simulink model "GFMGSP"  (R2022a)
settings: Solver=FixedStepAuto  StartTime=0.0  StopTime=3  FixedStep=Ts  RelTol=1e-3
values from neighbouring files (symbols this model uses):
  Cf1 = 0.002    [GFMGSP_Para.m]
  Cf2 = 0.2    [GFMGSP_Para.m]
  dt_jump = 2    [GFMGSP_Para.m]
  dt_sag = 0.01    [GFMGSP_Para.m]
  ki_pll1 = 0    [GFMGSP_Para.m]
  kp_pll1 = w_pll1    [GFMGSP_Para.m]
  Kq = Kq    [GFMGSP_Para.m]
  L1 = X1    [GFMGSP_Para.m]
  L2 = X2    [GFMGSP_Para.m]
  Lc1 = 1e-9    (= 1e-09)    [GFMGSP_Para.m]
  Lc2 = 1e-9    (= 1e-09)    [GFMGSP_Para.m]
  Lf1 = 0.1    [GFMGSP_Para.m]
  Lf2 = 0.1    [GFMGSP_Para.m]
  Lg = Xg    [GFMGSP_Para.m]
  M = Kgfm/Wbase    [GFMGSP_Para.m]
  phase_jump = -1.2    [GFMGSP_Para.m]
  Pm = Pref    [GFMGSP_Para.m]
  position = position    [GFMGSP_Para.m]
  R1 = R1    [GFMGSP_Para.m]
  R2 = R2    [GFMGSP_Para.m]
  Rg = Rg    [GFMGSP_Para.m]
  Sbase = 1    [GFMGSP_Para.m]
  Scale_ki_v = 60    [GFMGSP_Para.m]
  t0 = 2    [GFMGSP_Para.m]
  t0_jump = 10    [GFMGSP_Para.m]
  t0_sag = 10    [GFMGSP_Para.m]
  tc1 = t_c-0.002    [GFMGSP_Para.m]
  tc2 = t_c2    [GFMGSP_Para.m]
  tc3 = t_c3    [GFMGSP_Para.m]
  Ts = 1/Fs    (= 1e-05)    [GFMGSP_Para.m]
  v_sag = 0.1    [GFMGSP_Para.m]
  Vbase = 1    [GFMGSP_Para.m]
  w_droop = 15*2*pi    (= 94.2477796077)    [GFMGSP_Para.m]
  w_i_GFL1 = 1000 *2*pi    (= 6283.18530718)    [GFMGSP_Para.m]
  w_i_GFM = 2500*2*pi    (= 15707.9632679)    [GFMGSP_Para.m]
  w_pll1 = k1p    [GFMGSP_Para.m]
  w_tau1 = 1e3 *2*pi    (= 6283.18530718)    [GFMGSP_Para.m]
  w_tvc = 25*2*pi    (= 157.079632679)    [GFMGSP_Para.m]
  w_v_GFM = 200 *2*pi    (= 1256.63706144)    [GFMGSP_Para.m]
  Wbase = 2*pi*50    (= 314.159265359)    [GFMGSP_Para.m]
  Zbase = Vbase/Ibase    (= 1)    [GFMGSP_Para.m]
undefined symbols (not defined in the file or in its folder): DiscIntNeverNeededParam, I1d, I1q, initial, V1ref
libraries: spsVoltageMeasurementLib x114, spsCurrentMeasurementLib x93, spsThreePhaseSeriesRLCBranchLib x45, SimplexPS x42, spsControlledVoltageSourceLib x39, SimplexPS_2015a x14, spsGroundLib x10, spsSeriesRLCBranchLib x9, spsThreePhaseBreakerLib x6, spsMultimeterLib x3, spsThreePhaseFaultLib x3, spspowerguiLib x1
(part 3 of 7)

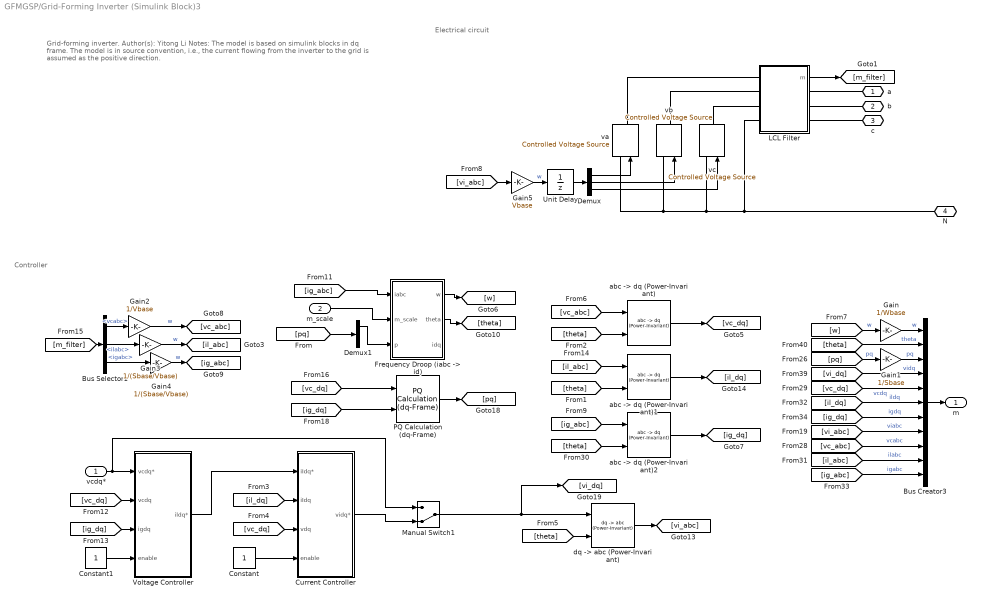
== system GFMGSP/Grid-Forming Inverter (Simulink Block)3 ==
  note: Grid-forming inverter.
      |
      | Author(s): Yitong Li
      |
      | Notes:
      |
      | The model is based on simulink blocks in dq frame.
      |
      | The model is in source convention, i.e., the current flowing from the inverter to the grid is assumed as the positive direction.
  note: Electrical circuit
  note: Controller
  vcdq* : Inport
  m_scale : Inport  Port=2
  Bus Creator3 : BusCreator  Inputs=11
  Bus Selector1 : BusSelector  OutputSignals=vcabc,ilabc,igabc
  Constant : Constant
  Constant1 : Constant
  Current Controller : Subsystem  mask{Ts=Ts, Wbase=Wbase, Lf=Lf/Wbase, Kg=0, Kp=w_i*Lf/Wbase, Ki=w_i*w_i/4*Lf/Wbase, xdmax=inf, xqmax=inf, Kcd=0}
      mask prompts: Ts "Sampling Time (s)"; Wbase "Base Angular Frequency (rad/s)"; Lf "Inductance"; Kg "Estimator Gain"; Kp "Proportional Gain"; Ki "Integral Gain"; xdmax "Voltage D Limit"; xqmax "Voltage Q Limit"; Kcd "Cross Decoupling Gain"
  Demux : Demux  Outputs=3
  Demux1 : Demux  Outputs=2
  "Frequency Droop (iabc -> id)" : Subsystem  AncestorBlock=|  mask{Ts=Ts, Sbase=Sbase, Vbase=Vbase, Wbase=Wbase, m=m, w_tau=w_droop, theta0=0, i0=Pm, w0=1}
      | SimplexPS/Frequency Droop
      | (iabc -> id)
      mask prompts: Ts "Ts (s), samping period"; Sbase "Sbase (VA), base power"; Vbase "Vbase (V), base voltage"; Wbase "Wbase (rad/s), base angular frequency"; m "m (pu), droop gain"; w_tau "w_tau (rad/s), low-pass filter bandwidth"; theta0 "theta0 (rad), initial angle"; i0 "i0 (pu), current setting point"; w0 "w0 (pu), frequency setting point"
  Gain : Gain  Gain=1/Wbase
  Gain1 : Gain  Gain=1/Sbase
  Gain2 : Gain  Gain=1/Vbase
  Gain3 : Gain  Gain=1/(Sbase/Vbase)
  Gain4 : Gain  Gain=1/(Sbase/Vbase)
  Gain5 : Gain  Gain=Vbase
  LCL Filter : Subsystem  AncestorBlock=SimplexPS/LCL Filter  mask{Lf=Lf*(Vbase^2/Sbase)/Wbase, Rf=1e-2*(Vbase^2/Sbase), Lc=Lc*(Vbase^2/Sbase)/Wbase, Rc=1e-9*(Vbase^2/Sbase), Cf=Cf*(Sbase/Vbase^2)/Wbase, Rd=1e-3*(Vbase^2/Sbase)}
      mask prompts: Lf "Lf (H)"; Rf "Rf (Ohm)"; Lc "Lc (H)"; Rc "Rc (Ohm)"; Cf "Cf (F)"; Rd "Rd (Ohm)"
  Manual Switch1 : ManualSwitch  CurrentSetting=0
  PQ Calculation (dq-Frame) : SimplexPS/PQ Calculation (dq-Frame)  SystemSampleTime=-1  VariantActivationTime=update diagram  Latency=0  AutoFrameSizeCalculation=off
      settings: SourceProductName=Simplex Power Systems
  Unit Delay : UnitDelay  SampleTime=-1  HasFrameUpgradeWarning=on
  Voltage Controller : Subsystem  mask{Ts=Ts, Wbase=Wbase, Cf=Cf/Wbase, Kg=0, Kp=w_v*Cf/Wbase, Ki=w_v*w_v/4*Cf/Wbase*Scale_ki_v, xdmax=inf, xqmax=inf, Kcd=0}
      mask prompts: Ts "Sampling Time (s)"; Wbase "Base Angular Frequency (rad/s)"; Cf "Capacitance"; Kg "Estimator Gain"; Kp "Proportional Gain"; Ki "Integral Gain"; xdmax "Current D Limit"; xqmax "Current Q Limit"; Kcd "Cross Decoupling Gain"
  "abc -> dq (Power-Invariant)" : SimplexPS/abc -> dq (Power-Invariant)  SystemSampleTime=-1  VariantActivationTime=update diagram  Latency=0  AutoFrameSizeCalculation=off
      settings: SourceProductName=Simplex Power Systems
  "abc -> dq (Power-Invariant)1" : SimplexPS/abc -> dq (Power-Invariant)  SystemSampleTime=-1  VariantActivationTime=update diagram  Latency=0  AutoFrameSizeCalculation=off
      settings: SourceProductName=Simplex Power Systems
  "abc -> dq (Power-Invariant)2" : SimplexPS/abc -> dq (Power-Invariant)  SystemSampleTime=-1  VariantActivationTime=update diagram  Latency=0  AutoFrameSizeCalculation=off
      settings: SourceProductName=Simplex Power Systems
  "dq -> abc (Power-Invariant)" : SimplexPS/dq -> abc (Power-Invariant)  SystemSampleTime=-1  VariantActivationTime=update diagram  Latency=0  AutoFrameSizeCalculation=off
      settings: SourceProductName=Simplex Power Systems
  va : spsControlledVoltageSourceLib/Controlled Voltage Source  Initialize=on  Source_Type=AC  Amplitude=0  Phase=0  Frequency=0  Measurements=None
  vb : spsControlledVoltageSourceLib/Controlled Voltage Source  Initialize=on  Source_Type=AC  Amplitude=0  Phase=0  Frequency=0  Measurements=None
  vc : spsControlledVoltageSourceLib/Controlled Voltage Source  Initialize=on  Source_Type=AC  Amplitude=0  Phase=0  Frequency=0  Measurements=None
  a : PMIOPort  Side=Right
  b : PMIOPort  Port=2  Side=Right
  c : PMIOPort  Port=3  Side=Right
  N : PMIOPort  Port=4  Side=Right
  m : Outport
  wires:
  [ig_dq] -> Voltage Controller/3(igdq)
  [vc_dq] -> Voltage Controller/2(vcdq)
  Constant1/1 -> Voltage Controller/4(enable)
  Voltage Controller/1(ildq*) -> Current Controller/1(iIdq*)
  vcdq*/1 -> Manual Switch1/1, Voltage Controller/1(vcdq*)
  [ig_abc] -> Bus Creator3/11  "igabc"
  [il_abc] -> Bus Creator3/10  "ilabc"
  [vc_abc] -> Bus Creator3/9  "vcabc"
  [vi_abc] -> Bus Creator3/8  "viabc"
  [ig_dq] -> Bus Creator3/7  "igdq"
  [il_dq] -> Bus Creator3/6  "ildq"
  [vc_dq] -> Bus Creator3/5  "vcdq"
  [vi_dq] -> Bus Creator3/4  "vidq"
  Gain1/1 -> Bus Creator3/3  "pq"
  [theta] -> Bus Creator3/2  "theta"
  Gain/1 -> Bus Creator3/1  "w"
  [pq] -> Gain1/1  "pq"
  [w] -> Gain/1  "w"
  "abc -> dq (Power-Invariant)1"/1 -> [il_dq]
  "abc -> dq (Power-Invariant)2"/1 -> [ig_dq]
  "abc -> dq (Power-Invariant)"/1 -> [vc_dq]
  [ig_abc] -> "Frequency Droop (iabc -> id)"/1(iabc)
  [il_dq] -> Current Controller/2(iIdq)
  [ig_dq] -> PQ Calculation (dq-Frame)/2
  PQ Calculation (dq-Frame)/1 -> [pq]
  [vc_dq] -> PQ Calculation (dq-Frame)/1
  [theta] -> "dq -> abc (Power-Invariant)"/2
  [vc_dq] -> Current Controller/3(vdq)
  Constant/1 -> Current Controller/4(enable)
  "Frequency Droop (iabc -> id)"/1(w) -> [w]
  "Frequency Droop (iabc -> id)"/2(theta) -> [theta]
  [theta] -> "abc -> dq (Power-Invariant)2"/2
  [ig_abc] -> "abc -> dq (Power-Invariant)2"/1
  [il_abc] -> "abc -> dq (Power-Invariant)1"/1
  [vc_abc] -> "abc -> dq (Power-Invariant)"/1
  [theta] -> "abc -> dq (Power-Invariant)1"/2
  [theta] -> "abc -> dq (Power-Invariant)"/2
  Demux/3 -> vc/1
  Demux/2 -> vb/1
  Demux/1 -> va/1
  LCL Filter/1(m) -> [m_filter]
  Bus Creator3/1 -> m/1
  "dq -> abc (Power-Invariant)"/1 -> [vi_abc]
  m_scale/1 -> "Frequency Droop (iabc -> id)"/2(m_scale)
  [vi_abc] -> Gain5/1
  Unit Delay/1 -> Demux/1
  Demux1/1 -> "Frequency Droop (iabc -> id)"/3(p)
  [pq] -> Demux1/1
  Bus Selector1/3 -> Gain4/1  "<igabc>"
  Bus Selector1/2 -> Gain3/1  "<ilabc>"
  Bus Selector1/1 -> Gain2/1  "<vcabc>"
  Gain4/1 -> [ig_abc]  "w"
  [m_filter] -> Bus Selector1/1
  Gain2/1 -> [vc_abc]  "w"
  Gain3/1 -> [il_abc]  "w"
  Gain5/1 -> Unit Delay/1  "w"
  Manual Switch1/1 -> [vi_dq], "dq -> abc (Power-Invariant)"/1
  Current Controller/1(vidq*) -> Manual Switch1/2
  connections:
  LCL Filter/LConn3 -- vc/RConn1
  va/LConn1 -- vb/LConn1 -- vc/LConn1 -- LCL Filter/LConn4 -- N/RConn1
  LCL Filter/RConn3 -- c/RConn1
  LCL Filter/RConn2 -- b/RConn1
  LCL Filter/RConn1 -- a/RConn1
  LCL Filter/LConn1 -- va/RConn1
  LCL Filter/LConn2 -- vb/RConn1

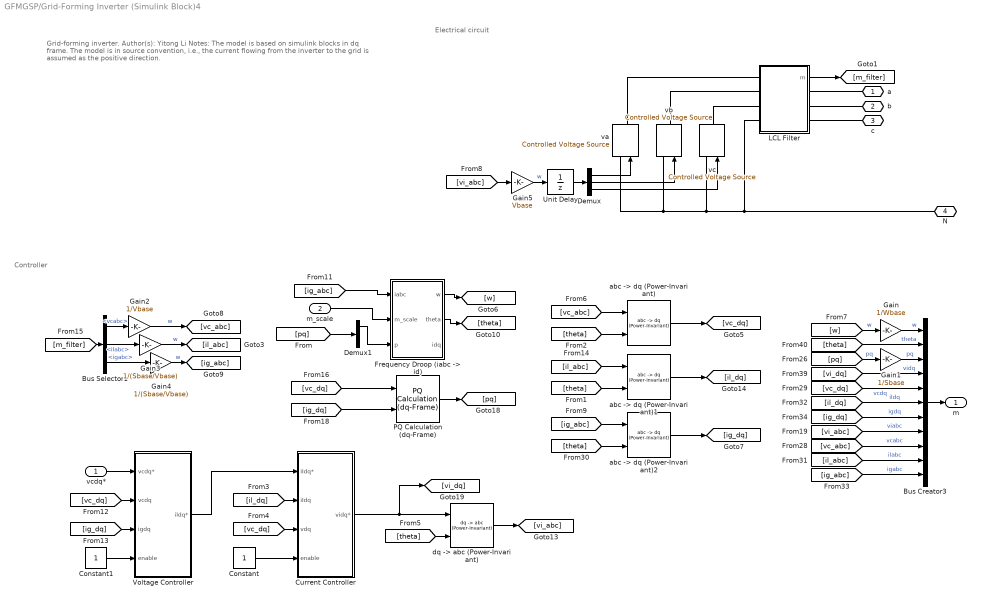
== system GFMGSP/Grid-Forming Inverter (Simulink Block)4 ==
  note: Grid-forming inverter.
      |
      | Author(s): Yitong Li
      |
      | Notes:
      |
      | The model is based on simulink blocks in dq frame.
      |
      | The model is in source convention, i.e., the current flowing from the inverter to the grid is assumed as the positive direction.
  note: Electrical circuit
  note: Controller
  vcdq* : Inport
  m_scale : Inport  Port=2
  Bus Creator3 : BusCreator  Inputs=11
  Bus Selector1 : BusSelector  OutputSignals=vcabc,ilabc,igabc
  Constant : Constant
  Constant1 : Constant
  Current Controller : Subsystem  mask{Ts=Ts, Wbase=Wbase, Lf=Lf/Wbase, Kg=0, Kp=w_i*Lf/Wbase, Ki=w_i*w_i/4*Lf/Wbase, xdmax=inf, xqmax=inf, Kcd=0}
      mask prompts: Ts "Sampling Time (s)"; Wbase "Base Angular Frequency (rad/s)"; Lf "Inductance"; Kg "Estimator Gain"; Kp "Proportional Gain"; Ki "Integral Gain"; xdmax "Voltage D Limit"; xqmax "Voltage Q Limit"; Kcd "Cross Decoupling Gain"
  Demux : Demux  Outputs=3
  Demux1 : Demux  Outputs=2
  "Frequency Droop (iabc -> id)" : Subsystem  AncestorBlock=|  mask{Ts=Ts, Sbase=Sbase, Vbase=Vbase, Wbase=Wbase, m=m, w_tau=w_droop, theta0=0, i0=Pm, w0=1}
      | SimplexPS/Frequency Droop
      | (iabc -> id)
      mask prompts: Ts "Ts (s), samping period"; Sbase "Sbase (VA), base power"; Vbase "Vbase (V), base voltage"; Wbase "Wbase (rad/s), base angular frequency"; m "m (pu), droop gain"; w_tau "w_tau (rad/s), low-pass filter bandwidth"; theta0 "theta0 (rad), initial angle"; i0 "i0 (pu), current setting point"; w0 "w0 (pu), frequency setting point"
  Gain : Gain  Gain=1/Wbase
  Gain1 : Gain  Gain=1/Sbase
  Gain2 : Gain  Gain=1/Vbase
  Gain3 : Gain  Gain=1/(Sbase/Vbase)
  Gain4 : Gain  Gain=1/(Sbase/Vbase)
  Gain5 : Gain  Gain=Vbase
  LCL Filter : Subsystem  AncestorBlock=SimplexPS/LCL Filter  mask{Lf=Lf*(Vbase^2/Sbase)/Wbase, Rf=1e-9*(Vbase^2/Sbase), Lc=Lc*(Vbase^2/Sbase)/Wbase, Rc=1e-9*(Vbase^2/Sbase), Cf=Cf*(Sbase/Vbase^2)/Wbase, Rd=1e-9*(Vbase^2/Sbase)}
      mask prompts: Lf "Lf (H)"; Rf "Rf (Ohm)"; Lc "Lc (H)"; Rc "Rc (Ohm)"; Cf "Cf (F)"; Rd "Rd (Ohm)"
  PQ Calculation (dq-Frame) : SimplexPS/PQ Calculation (dq-Frame)  SystemSampleTime=-1  VariantActivationTime=update diagram  Latency=0  AutoFrameSizeCalculation=off
      settings: SourceProductName=Simplex Power Systems
  Unit Delay : UnitDelay  SampleTime=-1  HasFrameUpgradeWarning=on
  Voltage Controller : Subsystem  mask{Ts=Ts, Wbase=Wbase, Cf=Cf/Wbase, Kg=0, Kp=w_v*Cf/Wbase, Ki=w_v*w_v/4*Cf/Wbase*Scale_ki_v, xdmax=inf, xqmax=inf, Kcd=0}
      mask prompts: Ts "Sampling Time (s)"; Wbase "Base Angular Frequency (rad/s)"; Cf "Capacitance"; Kg "Estimator Gain"; Kp "Proportional Gain"; Ki "Integral Gain"; xdmax "Current D Limit"; xqmax "Current Q Limit"; Kcd "Cross Decoupling Gain"
  "abc -> dq (Power-Invariant)" : SimplexPS/abc -> dq (Power-Invariant)  SystemSampleTime=-1  VariantActivationTime=update diagram  Latency=0  AutoFrameSizeCalculation=off
      settings: SourceProductName=Simplex Power Systems
  "abc -> dq (Power-Invariant)1" : SimplexPS/abc -> dq (Power-Invariant)  SystemSampleTime=-1  VariantActivationTime=update diagram  Latency=0  AutoFrameSizeCalculation=off
      settings: SourceProductName=Simplex Power Systems
  "abc -> dq (Power-Invariant)2" : SimplexPS/abc -> dq (Power-Invariant)  SystemSampleTime=-1  VariantActivationTime=update diagram  Latency=0  AutoFrameSizeCalculation=off
      settings: SourceProductName=Simplex Power Systems
  "dq -> abc (Power-Invariant)" : SimplexPS/dq -> abc (Power-Invariant)  SystemSampleTime=-1  VariantActivationTime=update diagram  Latency=0  AutoFrameSizeCalculation=off
      settings: SourceProductName=Simplex Power Systems
  va : spsControlledVoltageSourceLib/Controlled Voltage Source  Initialize=on  Source_Type=AC  Amplitude=0  Phase=0  Frequency=0  Measurements=None
  vb : spsControlledVoltageSourceLib/Controlled Voltage Source  Initialize=on  Source_Type=AC  Amplitude=0  Phase=0  Frequency=0  Measurements=None
  vc : spsControlledVoltageSourceLib/Controlled Voltage Source  Initialize=on  Source_Type=AC  Amplitude=0  Phase=0  Frequency=0  Measurements=None
  a : PMIOPort  Side=Right
  b : PMIOPort  Port=2  Side=Right
  c : PMIOPort  Port=3  Side=Right
  N : PMIOPort  Port=4  Side=Right
  m : Outport
  wires:
  [ig_dq] -> Voltage Controller/3(igdq)
  [vc_dq] -> Voltage Controller/2(vcdq)
  Constant1/1 -> Voltage Controller/4(enable)
  Voltage Controller/1(ildq*) -> Current Controller/1(iIdq*)
  vcdq*/1 -> Voltage Controller/1(vcdq*)
  [ig_abc] -> Bus Creator3/11  "igabc"
  [il_abc] -> Bus Creator3/10  "ilabc"
  [vc_abc] -> Bus Creator3/9  "vcabc"
  [vi_abc] -> Bus Creator3/8  "viabc"
  [ig_dq] -> Bus Creator3/7  "igdq"
  [il_dq] -> Bus Creator3/6  "ildq"
  [vc_dq] -> Bus Creator3/5  "vcdq"
  [vi_dq] -> Bus Creator3/4  "vidq"
  Gain1/1 -> Bus Creator3/3  "pq"
  [theta] -> Bus Creator3/2  "theta"
  Gain/1 -> Bus Creator3/1  "w"
  [pq] -> Gain1/1  "pq"
  [w] -> Gain/1  "w"
  "abc -> dq (Power-Invariant)1"/1 -> [il_dq]
  "abc -> dq (Power-Invariant)2"/1 -> [ig_dq]
  "abc -> dq (Power-Invariant)"/1 -> [vc_dq]
  [ig_abc] -> "Frequency Droop (iabc -> id)"/1(iabc)
  [il_dq] -> Current Controller/2(iIdq)
  [ig_dq] -> PQ Calculation (dq-Frame)/2
  PQ Calculation (dq-Frame)/1 -> [pq]
  [vc_dq] -> PQ Calculation (dq-Frame)/1
  [theta] -> "dq -> abc (Power-Invariant)"/2
  Current Controller/1(vidq*) -> "dq -> abc (Power-Invariant)"/1, [vi_dq]
  [vc_dq] -> Current Controller/3(vdq)
  Constant/1 -> Current Controller/4(enable)
  "Frequency Droop (iabc -> id)"/1(w) -> [w]
  "Frequency Droop (iabc -> id)"/2(theta) -> [theta]
  [theta] -> "abc -> dq (Power-Invariant)2"/2
  [ig_abc] -> "abc -> dq (Power-Invariant)2"/1
  [il_abc] -> "abc -> dq (Power-Invariant)1"/1
  [vc_abc] -> "abc -> dq (Power-Invariant)"/1
  [theta] -> "abc -> dq (Power-Invariant)1"/2
  [theta] -> "abc -> dq (Power-Invariant)"/2
  Demux/3 -> vc/1
  Demux/2 -> vb/1
  Demux/1 -> va/1
  LCL Filter/1(m) -> [m_filter]
  Bus Creator3/1 -> m/1
  "dq -> abc (Power-Invariant)"/1 -> [vi_abc]
  m_scale/1 -> "Frequency Droop (iabc -> id)"/2(m_scale)
  [vi_abc] -> Gain5/1
  Unit Delay/1 -> Demux/1
  Demux1/1 -> "Frequency Droop (iabc -> id)"/3(p)
  [pq] -> Demux1/1
  Bus Selector1/3 -> Gain4/1  "<igabc>"
  Bus Selector1/2 -> Gain3/1  "<ilabc>"
  Bus Selector1/1 -> Gain2/1  "<vcabc>"
  Gain4/1 -> [ig_abc]  "w"
  [m_filter] -> Bus Selector1/1
  Gain2/1 -> [vc_abc]  "w"
  Gain3/1 -> [il_abc]  "w"
  Gain5/1 -> Unit Delay/1  "w"
  connections:
  LCL Filter/LConn3 -- vc/RConn1
  va/LConn1 -- vb/LConn1 -- vc/LConn1 -- LCL Filter/LConn4 -- N/RConn1
  LCL Filter/RConn3 -- c/RConn1
  LCL Filter/RConn2 -- b/RConn1
  LCL Filter/RConn1 -- a/RConn1
  LCL Filter/LConn1 -- va/RConn1
  LCL Filter/LConn2 -- vb/RConn1

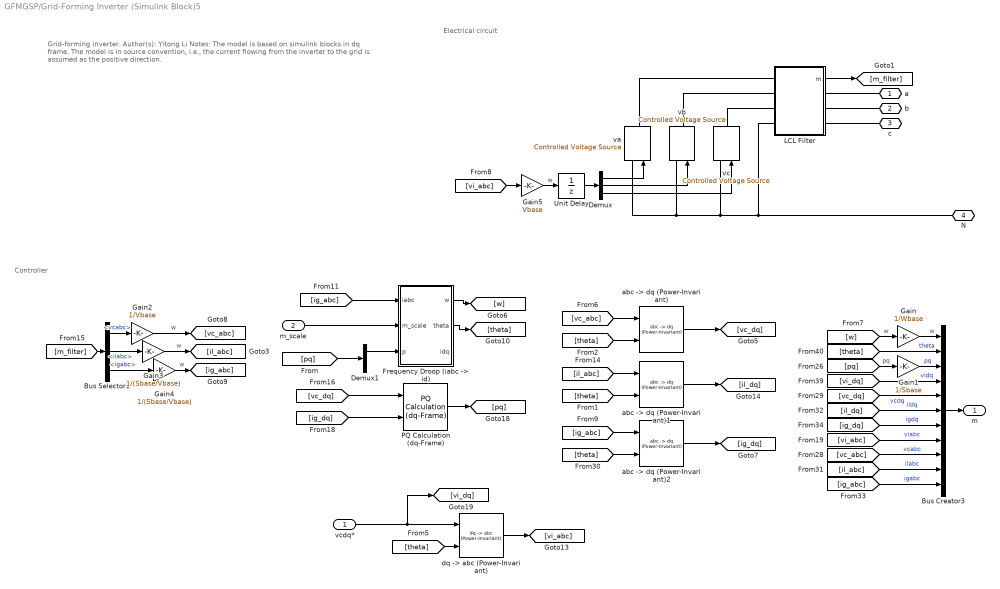
== system GFMGSP/Grid-Forming Inverter (Simulink Block)5 ==
  note: Grid-forming inverter.
      |
      | Author(s): Yitong Li
      |
      | Notes:
      |
      | The model is based on simulink blocks in dq frame.
      |
      | The model is in source convention, i.e., the current flowing from the inverter to the grid is assumed as the positive direction.
  note: Electrical circuit
  note: Controller
  vcdq* : Inport
  m_scale : Inport  Port=2
  Bus Creator3 : BusCreator  Inputs=11
  Bus Selector1 : BusSelector  OutputSignals=vcabc,ilabc,igabc
  Demux : Demux  Outputs=3
  Demux1 : Demux  Outputs=2
  "Frequency Droop (iabc -> id)" : Subsystem  AncestorBlock=|  mask{Ts=Ts, Sbase=Sbase, Vbase=Vbase, Wbase=Wbase, m=m, w_tau=w_droop, theta0=0, i0=Pm, w0=1}
      | SimplexPS/Frequency Droop
      | (iabc -> id)
      mask prompts: Ts "Ts (s), samping period"; Sbase "Sbase (VA), base power"; Vbase "Vbase (V), base voltage"; Wbase "Wbase (rad/s), base angular frequency"; m "m (pu), droop gain"; w_tau "w_tau (rad/s), low-pass filter bandwidth"; theta0 "theta0 (rad), initial angle"; i0 "i0 (pu), current setting point"; w0 "w0 (pu), frequency setting point"
  Gain : Gain  Gain=1/Wbase
  Gain1 : Gain  Gain=1/Sbase
  Gain2 : Gain  Gain=1/Vbase
  Gain3 : Gain  Gain=1/(Sbase/Vbase)
  Gain4 : Gain  Gain=1/(Sbase/Vbase)
  Gain5 : Gain  Gain=Vbase
  LCL Filter : Subsystem  AncestorBlock=SimplexPS/LCL Filter  mask{Lf=Lf*(Vbase^2/Sbase)/Wbase, Rf=1e-2*(Vbase^2/Sbase), Lc=Lc*(Vbase^2/Sbase)/Wbase, Rc=1e-6*(Vbase^2/Sbase), Cf=Cf*(Sbase/Vbase^2)/Wbase, Rd=1e-6*(Vbase^2/Sbase)}
      mask prompts: Lf "Lf (H)"; Rf "Rf (Ohm)"; Lc "Lc (H)"; Rc "Rc (Ohm)"; Cf "Cf (F)"; Rd "Rd (Ohm)"
  PQ Calculation (dq-Frame) : SimplexPS/PQ Calculation (dq-Frame)  SystemSampleTime=-1  VariantActivationTime=update diagram  Latency=0  AutoFrameSizeCalculation=off
      settings: SourceProductName=Simplex Power Systems
  Unit Delay : UnitDelay  SampleTime=-1  HasFrameUpgradeWarning=on
  "abc -> dq (Power-Invariant)" : SimplexPS/abc -> dq (Power-Invariant)  SystemSampleTime=-1  VariantActivationTime=update diagram  Latency=0  AutoFrameSizeCalculation=off
      settings: SourceProductName=Simplex Power Systems
  "abc -> dq (Power-Invariant)1" : SimplexPS/abc -> dq (Power-Invariant)  SystemSampleTime=-1  VariantActivationTime=update diagram  Latency=0  AutoFrameSizeCalculation=off
      settings: SourceProductName=Simplex Power Systems
  "abc -> dq (Power-Invariant)2" : SimplexPS/abc -> dq (Power-Invariant)  SystemSampleTime=-1  VariantActivationTime=update diagram  Latency=0  AutoFrameSizeCalculation=off
      settings: SourceProductName=Simplex Power Systems
  "dq -> abc (Power-Invariant)" : SimplexPS/dq -> abc (Power-Invariant)  SystemSampleTime=-1  VariantActivationTime=update diagram  Latency=0  AutoFrameSizeCalculation=off
      settings: SourceProductName=Simplex Power Systems
  va : spsControlledVoltageSourceLib/Controlled Voltage Source  Initialize=on  Source_Type=AC  Amplitude=0  Phase=0  Frequency=0  Measurements=None
  vb : spsControlledVoltageSourceLib/Controlled Voltage Source  Initialize=on  Source_Type=AC  Amplitude=0  Phase=0  Frequency=0  Measurements=None
  vc : spsControlledVoltageSourceLib/Controlled Voltage Source  Initialize=on  Source_Type=AC  Amplitude=0  Phase=0  Frequency=0  Measurements=None
  a : PMIOPort  Side=Right
  b : PMIOPort  Port=2  Side=Right
  c : PMIOPort  Port=3  Side=Right
  N : PMIOPort  Port=4  Side=Right
  m : Outport
  wires:
  [ig_abc] -> Bus Creator3/11  "igabc"
  [il_abc] -> Bus Creator3/10  "ilabc"
  [vc_abc] -> Bus Creator3/9  "vcabc"
  [vi_abc] -> Bus Creator3/8  "viabc"
  [ig_dq] -> Bus Creator3/7  "igdq"
  [il_dq] -> Bus Creator3/6  "ildq"
  [vc_dq] -> Bus Creator3/5  "vcdq"
  [vi_dq] -> Bus Creator3/4  "vidq"
  Gain1/1 -> Bus Creator3/3  "pq"
  [theta] -> Bus Creator3/2  "theta"
  Gain/1 -> Bus Creator3/1  "w"
  [pq] -> Gain1/1  "pq"
  [w] -> Gain/1  "w"
  "abc -> dq (Power-Invariant)1"/1 -> [il_dq]
  "abc -> dq (Power-Invariant)2"/1 -> [ig_dq]
  "abc -> dq (Power-Invariant)"/1 -> [vc_dq]
  [ig_abc] -> "Frequency Droop (iabc -> id)"/1(iabc)
  [ig_dq] -> PQ Calculation (dq-Frame)/2
  PQ Calculation (dq-Frame)/1 -> [pq]
  [vc_dq] -> PQ Calculation (dq-Frame)/1
  [theta] -> "dq -> abc (Power-Invariant)"/2
  vcdq*/1 -> "dq -> abc (Power-Invariant)"/1, [vi_dq]
  "Frequency Droop (iabc -> id)"/1(w) -> [w]
  "Frequency Droop (iabc -> id)"/2(theta) -> [theta]
  [theta] -> "abc -> dq (Power-Invariant)2"/2
  [ig_abc] -> "abc -> dq (Power-Invariant)2"/1
  [il_abc] -> "abc -> dq (Power-Invariant)1"/1
  [vc_abc] -> "abc -> dq (Power-Invariant)"/1
  [theta] -> "abc -> dq (Power-Invariant)1"/2
  [theta] -> "abc -> dq (Power-Invariant)"/2
  Demux/3 -> vc/1
  Demux/2 -> vb/1
  Demux/1 -> va/1
  LCL Filter/1(m) -> [m_filter]
  Bus Creator3/1 -> m/1
  "dq -> abc (Power-Invariant)"/1 -> [vi_abc]
  m_scale/1 -> "Frequency Droop (iabc -> id)"/2(m_scale)
  [vi_abc] -> Gain5/1
  Unit Delay/1 -> Demux/1
  Demux1/1 -> "Frequency Droop (iabc -> id)"/3(p)
  [pq] -> Demux1/1
  Bus Selector1/3 -> Gain4/1  "<igabc>"
  Bus Selector1/2 -> Gain3/1  "<ilabc>"
  Bus Selector1/1 -> Gain2/1  "<vcabc>"
  Gain4/1 -> [ig_abc]  "w"
  [m_filter] -> Bus Selector1/1
  Gain2/1 -> [vc_abc]  "w"
  Gain3/1 -> [il_abc]  "w"
  Gain5/1 -> Unit Delay/1  "w"
  connections:
  LCL Filter/LConn3 -- vc/RConn1
  va/LConn1 -- vb/LConn1 -- vc/LConn1 -- LCL Filter/LConn4 -- N/RConn1
  LCL Filter/RConn3 -- c/RConn1
  LCL Filter/RConn2 -- b/RConn1
  LCL Filter/RConn1 -- a/RConn1
  LCL Filter/LConn1 -- va/RConn1
  LCL Filter/LConn2 -- vb/RConn1

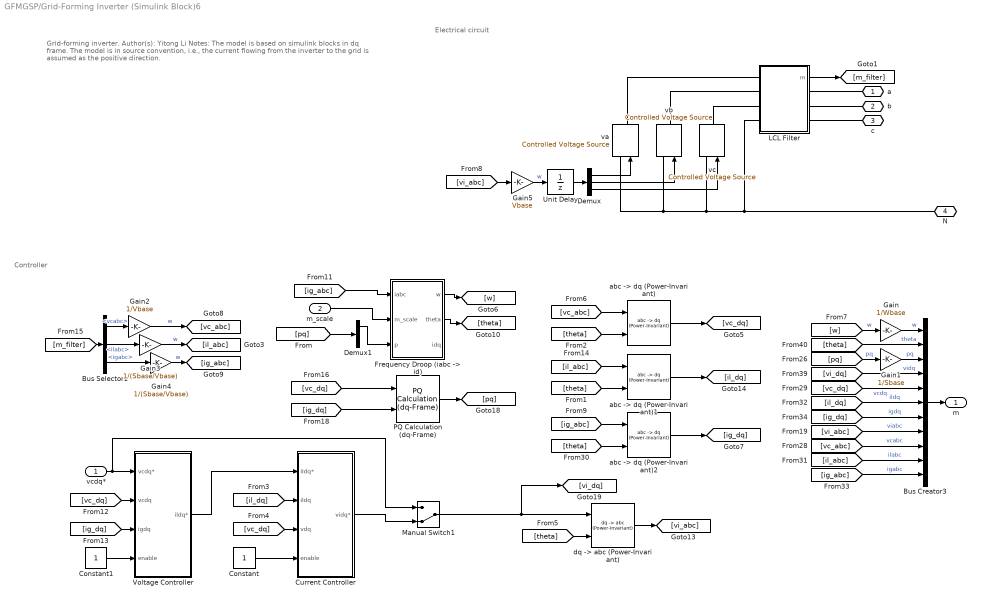
== system GFMGSP/Grid-Forming Inverter (Simulink Block)6 ==
  note: Grid-forming inverter.
      |
      | Author(s): Yitong Li
      |
      | Notes:
      |
      | The model is based on simulink blocks in dq frame.
      |
      | The model is in source convention, i.e., the current flowing from the inverter to the grid is assumed as the positive direction.
  note: Electrical circuit
  note: Controller
  vcdq* : Inport
  m_scale : Inport  Port=2
  Bus Creator3 : BusCreator  Inputs=11
  Bus Selector1 : BusSelector  OutputSignals=vcabc,ilabc,igabc
  Constant : Constant
  Constant1 : Constant
  Current Controller : Subsystem  mask{Ts=Ts, Wbase=Wbase, Lf=Lf/Wbase, Kg=0, Kp=w_i*Lf/Wbase, Ki=w_i*w_i/4*Lf/Wbase, xdmax=inf, xqmax=inf, Kcd=0}
      mask prompts: Ts "Sampling Time (s)"; Wbase "Base Angular Frequency (rad/s)"; Lf "Inductance"; Kg "Estimator Gain"; Kp "Proportional Gain"; Ki "Integral Gain"; xdmax "Voltage D Limit"; xqmax "Voltage Q Limit"; Kcd "Cross Decoupling Gain"
  Demux : Demux  Outputs=3
  Demux1 : Demux  Outputs=2
  "Frequency Droop (iabc -> id)" : Subsystem  AncestorBlock=|  mask{Ts=Ts, Sbase=Sbase, Vbase=Vbase, Wbase=Wbase, m=m, w_tau=w_droop, theta0=0, i0=Pm, w0=1}
      | SimplexPS/Frequency Droop
      | (iabc -> id)
      mask prompts: Ts "Ts (s), samping period"; Sbase "Sbase (VA), base power"; Vbase "Vbase (V), base voltage"; Wbase "Wbase (rad/s), base angular frequency"; m "m (pu), droop gain"; w_tau "w_tau (rad/s), low-pass filter bandwidth"; theta0 "theta0 (rad), initial angle"; i0 "i0 (pu), current setting point"; w0 "w0 (pu), frequency setting point"
  Gain : Gain  Gain=1/Wbase
  Gain1 : Gain  Gain=1/Sbase
  Gain2 : Gain  Gain=1/Vbase
  Gain3 : Gain  Gain=1/(Sbase/Vbase)
  Gain4 : Gain  Gain=1/(Sbase/Vbase)
  Gain5 : Gain  Gain=Vbase
  LCL Filter : Subsystem  AncestorBlock=SimplexPS/LCL Filter  mask{Lf=Lf*(Vbase^2/Sbase)/Wbase, Rf=1e-2*(Vbase^2/Sbase), Lc=Lc*(Vbase^2/Sbase)/Wbase, Rc=1e-9*(Vbase^2/Sbase), Cf=Cf*(Sbase/Vbase^2)/Wbase, Rd=1e-3*(Vbase^2/Sbase)}
      mask prompts: Lf "Lf (H)"; Rf "Rf (Ohm)"; Lc "Lc (H)"; Rc "Rc (Ohm)"; Cf "Cf (F)"; Rd "Rd (Ohm)"
  Manual Switch1 : ManualSwitch  CurrentSetting=0
  PQ Calculation (dq-Frame) : SimplexPS/PQ Calculation (dq-Frame)  SystemSampleTime=-1  VariantActivationTime=update diagram  Latency=0  AutoFrameSizeCalculation=off
      settings: SourceProductName=Simplex Power Systems
  Unit Delay : UnitDelay  SampleTime=-1  HasFrameUpgradeWarning=on
  Voltage Controller : Subsystem  mask{Ts=Ts, Wbase=Wbase, Cf=Cf/Wbase, Kg=0, Kp=w_v*Cf/Wbase, Ki=w_v*w_v/4*Cf/Wbase*Scale_ki_v, xdmax=inf, xqmax=inf, Kcd=0}
      mask prompts: Ts "Sampling Time (s)"; Wbase "Base Angular Frequency (rad/s)"; Cf "Capacitance"; Kg "Estimator Gain"; Kp "Proportional Gain"; Ki "Integral Gain"; xdmax "Current D Limit"; xqmax "Current Q Limit"; Kcd "Cross Decoupling Gain"
  "abc -> dq (Power-Invariant)" : SimplexPS/abc -> dq (Power-Invariant)  SystemSampleTime=-1  VariantActivationTime=update diagram  Latency=0  AutoFrameSizeCalculation=off
      settings: SourceProductName=Simplex Power Systems
  "abc -> dq (Power-Invariant)1" : SimplexPS/abc -> dq (Power-Invariant)  SystemSampleTime=-1  VariantActivationTime=update diagram  Latency=0  AutoFrameSizeCalculation=off
      settings: SourceProductName=Simplex Power Systems
  "abc -> dq (Power-Invariant)2" : SimplexPS/abc -> dq (Power-Invariant)  SystemSampleTime=-1  VariantActivationTime=update diagram  Latency=0  AutoFrameSizeCalculation=off
      settings: SourceProductName=Simplex Power Systems
  "dq -> abc (Power-Invariant)" : SimplexPS/dq -> abc (Power-Invariant)  SystemSampleTime=-1  VariantActivationTime=update diagram  Latency=0  AutoFrameSizeCalculation=off
      settings: SourceProductName=Simplex Power Systems
  va : spsControlledVoltageSourceLib/Controlled Voltage Source  Initialize=on  Source_Type=AC  Amplitude=0  Phase=0  Frequency=0  Measurements=None
  vb : spsControlledVoltageSourceLib/Controlled Voltage Source  Initialize=on  Source_Type=AC  Amplitude=0  Phase=0  Frequency=0  Measurements=None
  vc : spsControlledVoltageSourceLib/Controlled Voltage Source  Initialize=on  Source_Type=AC  Amplitude=0  Phase=0  Frequency=0  Measurements=None
  a : PMIOPort  Side=Right
  b : PMIOPort  Port=2  Side=Right
  c : PMIOPort  Port=3  Side=Right
  N : PMIOPort  Port=4  Side=Right
  m : Outport
  wires:
  [ig_dq] -> Voltage Controller/3(igdq)
  [vc_dq] -> Voltage Controller/2(vcdq)
  Constant1/1 -> Voltage Controller/4(enable)
  Voltage Controller/1(ildq*) -> Current Controller/1(iIdq*)
  vcdq*/1 -> Manual Switch1/1, Voltage Controller/1(vcdq*)
  [ig_abc] -> Bus Creator3/11  "igabc"
  [il_abc] -> Bus Creator3/10  "ilabc"
  [vc_abc] -> Bus Creator3/9  "vcabc"
  [vi_abc] -> Bus Creator3/8  "viabc"
  [ig_dq] -> Bus Creator3/7  "igdq"
  [il_dq] -> Bus Creator3/6  "ildq"
  [vc_dq] -> Bus Creator3/5  "vcdq"
  [vi_dq] -> Bus Creator3/4  "vidq"
  Gain1/1 -> Bus Creator3/3  "pq"
  [theta] -> Bus Creator3/2  "theta"
  Gain/1 -> Bus Creator3/1  "w"
  [pq] -> Gain1/1  "pq"
  [w] -> Gain/1  "w"
  "abc -> dq (Power-Invariant)1"/1 -> [il_dq]
  "abc -> dq (Power-Invariant)2"/1 -> [ig_dq]
  "abc -> dq (Power-Invariant)"/1 -> [vc_dq]
  [ig_abc] -> "Frequency Droop (iabc -> id)"/1(iabc)
  [il_dq] -> Current Controller/2(iIdq)
  [ig_dq] -> PQ Calculation (dq-Frame)/2
  PQ Calculation (dq-Frame)/1 -> [pq]
  [vc_dq] -> PQ Calculation (dq-Frame)/1
  [theta] -> "dq -> abc (Power-Invariant)"/2
  [vc_dq] -> Current Controller/3(vdq)
  Constant/1 -> Current Controller/4(enable)
  "Frequency Droop (iabc -> id)"/1(w) -> [w]
  "Frequency Droop (iabc -> id)"/2(theta) -> [theta]
  [theta] -> "abc -> dq (Power-Invariant)2"/2
  [ig_abc] -> "abc -> dq (Power-Invariant)2"/1
  [il_abc] -> "abc -> dq (Power-Invariant)1"/1
  [vc_abc] -> "abc -> dq (Power-Invariant)"/1
  [theta] -> "abc -> dq (Power-Invariant)1"/2
  [theta] -> "abc -> dq (Power-Invariant)"/2
  Demux/3 -> vc/1
  Demux/2 -> vb/1
  Demux/1 -> va/1
  LCL Filter/1(m) -> [m_filter]
  Bus Creator3/1 -> m/1
  "dq -> abc (Power-Invariant)"/1 -> [vi_abc]
  m_scale/1 -> "Frequency Droop (iabc -> id)"/2(m_scale)
  [vi_abc] -> Gain5/1
  Unit Delay/1 -> Demux/1
  Demux1/1 -> "Frequency Droop (iabc -> id)"/3(p)
  [pq] -> Demux1/1
  Bus Selector1/3 -> Gain4/1  "<igabc>"
  Bus Selector1/2 -> Gain3/1  "<ilabc>"
  Bus Selector1/1 -> Gain2/1  "<vcabc>"
  Gain4/1 -> [ig_abc]  "w"
  [m_filter] -> Bus Selector1/1
  Gain2/1 -> [vc_abc]  "w"
  Gain3/1 -> [il_abc]  "w"
  Gain5/1 -> Unit Delay/1  "w"
  Manual Switch1/1 -> [vi_dq], "dq -> abc (Power-Invariant)"/1
  Current Controller/1(vidq*) -> Manual Switch1/2
  connections:
  LCL Filter/LConn3 -- vc/RConn1
  va/LConn1 -- vb/LConn1 -- vc/LConn1 -- LCL Filter/LConn4 -- N/RConn1
  LCL Filter/RConn3 -- c/RConn1
  LCL Filter/RConn2 -- b/RConn1
  LCL Filter/RConn1 -- a/RConn1
  LCL Filter/LConn1 -- va/RConn1
  LCL Filter/LConn2 -- vb/RConn1

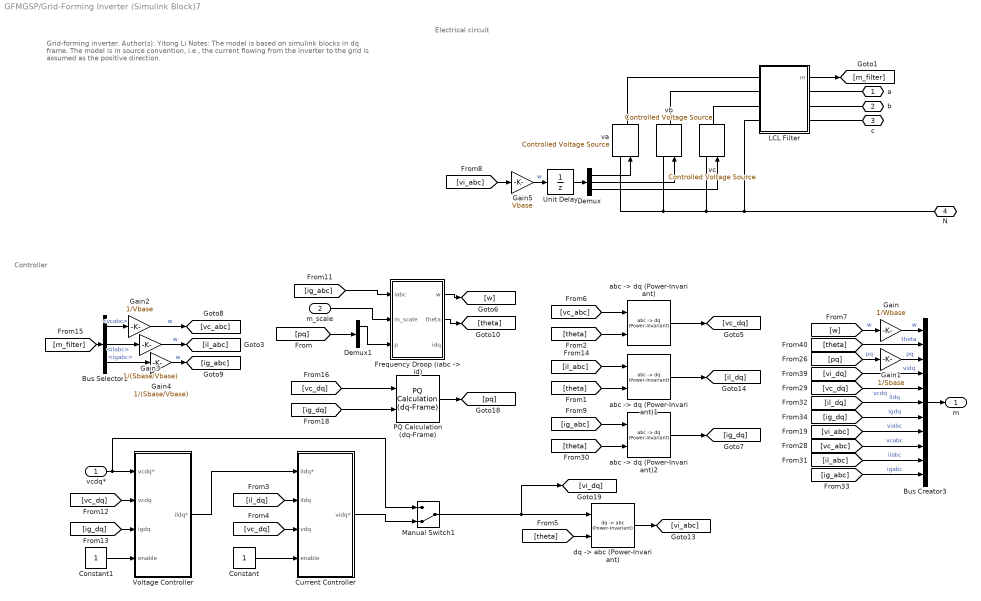
== system GFMGSP/Grid-Forming Inverter (Simulink Block)7 ==
  note: Grid-forming inverter.
      |
      | Author(s): Yitong Li
      |
      | Notes:
      |
      | The model is based on simulink blocks in dq frame.
      |
      | The model is in source convention, i.e., the current flowing from the inverter to the grid is assumed as the positive direction.
  note: Electrical circuit
  note: Controller
  vcdq* : Inport
  m_scale : Inport  Port=2
  Bus Creator3 : BusCreator  Inputs=11
  Bus Selector1 : BusSelector  OutputSignals=vcabc,ilabc,igabc
  Constant : Constant
  Constant1 : Constant
  Current Controller : Subsystem  mask{Ts=Ts, Wbase=Wbase, Lf=Lf/Wbase, Kg=0, Kp=w_i*Lf/Wbase, Ki=w_i*w_i/4*Lf/Wbase, xdmax=inf, xqmax=inf, Kcd=0}
      mask prompts: Ts "Sampling Time (s)"; Wbase "Base Angular Frequency (rad/s)"; Lf "Inductance"; Kg "Estimator Gain"; Kp "Proportional Gain"; Ki "Integral Gain"; xdmax "Voltage D Limit"; xqmax "Voltage Q Limit"; Kcd "Cross Decoupling Gain"
  Demux : Demux  Outputs=3
  Demux1 : Demux  Outputs=2
  "Frequency Droop (iabc -> id)" : Subsystem  AncestorBlock=|  mask{Ts=Ts, Sbase=Sbase, Vbase=Vbase, Wbase=Wbase, m=m, w_tau=w_droop, theta0=0, i0=Pm, w0=1}
      | SimplexPS/Frequency Droop
      | (iabc -> id)
      mask prompts: Ts "Ts (s), samping period"; Sbase "Sbase (VA), base power"; Vbase "Vbase (V), base voltage"; Wbase "Wbase (rad/s), base angular frequency"; m "m (pu), droop gain"; w_tau "w_tau (rad/s), low-pass filter bandwidth"; theta0 "theta0 (rad), initial angle"; i0 "i0 (pu), current setting point"; w0 "w0 (pu), frequency setting point"
  Gain : Gain  Gain=1/Wbase
  Gain1 : Gain  Gain=1/Sbase
  Gain2 : Gain  Gain=1/Vbase
  Gain3 : Gain  Gain=1/(Sbase/Vbase)
  Gain4 : Gain  Gain=1/(Sbase/Vbase)
  Gain5 : Gain  Gain=Vbase
  LCL Filter : Subsystem  AncestorBlock=SimplexPS/LCL Filter  mask{Lf=Lf*(Vbase^2/Sbase)/Wbase, Rf=1e-2*(Vbase^2/Sbase), Lc=Lc*(Vbase^2/Sbase)/Wbase, Rc=1e-9*(Vbase^2/Sbase), Cf=Cf*(Sbase/Vbase^2)/Wbase, Rd=1e-3*(Vbase^2/Sbase)}
      mask prompts: Lf "Lf (H)"; Rf "Rf (Ohm)"; Lc "Lc (H)"; Rc "Rc (Ohm)"; Cf "Cf (F)"; Rd "Rd (Ohm)"
  Manual Switch1 : ManualSwitch  CurrentSetting=0
  PQ Calculation (dq-Frame) : SimplexPS/PQ Calculation (dq-Frame)  SystemSampleTime=-1  VariantActivationTime=update diagram  Latency=0  AutoFrameSizeCalculation=off
      settings: SourceProductName=Simplex Power Systems
  Unit Delay : UnitDelay  SampleTime=-1  HasFrameUpgradeWarning=on
  Voltage Controller : Subsystem  mask{Ts=Ts, Wbase=Wbase, Cf=Cf/Wbase, Kg=0, Kp=w_v*Cf/Wbase, Ki=w_v*w_v/4*Cf/Wbase*Scale_ki_v, xdmax=inf, xqmax=inf, Kcd=0}
      mask prompts: Ts "Sampling Time (s)"; Wbase "Base Angular Frequency (rad/s)"; Cf "Capacitance"; Kg "Estimator Gain"; Kp "Proportional Gain"; Ki "Integral Gain"; xdmax "Current D Limit"; xqmax "Current Q Limit"; Kcd "Cross Decoupling Gain"
  "abc -> dq (Power-Invariant)" : SimplexPS/abc -> dq (Power-Invariant)  SystemSampleTime=-1  VariantActivationTime=update diagram  Latency=0  AutoFrameSizeCalculation=off
      settings: SourceProductName=Simplex Power Systems
  "abc -> dq (Power-Invariant)1" : SimplexPS/abc -> dq (Power-Invariant)  SystemSampleTime=-1  VariantActivationTime=update diagram  Latency=0  AutoFrameSizeCalculation=off
      settings: SourceProductName=Simplex Power Systems
  "abc -> dq (Power-Invariant)2" : SimplexPS/abc -> dq (Power-Invariant)  SystemSampleTime=-1  VariantActivationTime=update diagram  Latency=0  AutoFrameSizeCalculation=off
      settings: SourceProductName=Simplex Power Systems
  "dq -> abc (Power-Invariant)" : SimplexPS/dq -> abc (Power-Invariant)  SystemSampleTime=-1  VariantActivationTime=update diagram  Latency=0  AutoFrameSizeCalculation=off
      settings: SourceProductName=Simplex Power Systems
  va : spsControlledVoltageSourceLib/Controlled Voltage Source  Initialize=on  Source_Type=AC  Amplitude=0  Phase=0  Frequency=0  Measurements=None
  vb : spsControlledVoltageSourceLib/Controlled Voltage Source  Initialize=on  Source_Type=AC  Amplitude=0  Phase=0  Frequency=0  Measurements=None
  vc : spsControlledVoltageSourceLib/Controlled Voltage Source  Initialize=on  Source_Type=AC  Amplitude=0  Phase=0  Frequency=0  Measurements=None
  a : PMIOPort  Side=Right
  b : PMIOPort  Port=2  Side=Right
  c : PMIOPort  Port=3  Side=Right
  N : PMIOPort  Port=4  Side=Right
  m : Outport
  wires:
  [ig_dq] -> Voltage Controller/3(igdq)
  [vc_dq] -> Voltage Controller/2(vcdq)
  Constant1/1 -> Voltage Controller/4(enable)
  Voltage Controller/1(ildq*) -> Current Controller/1(iIdq*)
  vcdq*/1 -> Manual Switch1/1, Voltage Controller/1(vcdq*)
  [ig_abc] -> Bus Creator3/11  "igabc"
  [il_abc] -> Bus Creator3/10  "ilabc"
  [vc_abc] -> Bus Creator3/9  "vcabc"
  [vi_abc] -> Bus Creator3/8  "viabc"
  [ig_dq] -> Bus Creator3/7  "igdq"
  [il_dq] -> Bus Creator3/6  "ildq"
  [vc_dq] -> Bus Creator3/5  "vcdq"
  [vi_dq] -> Bus Creator3/4  "vidq"
  Gain1/1 -> Bus Creator3/3  "pq"
  [theta] -> Bus Creator3/2  "theta"
  Gain/1 -> Bus Creator3/1  "w"
  [pq] -> Gain1/1  "pq"
  [w] -> Gain/1  "w"
  "abc -> dq (Power-Invariant)1"/1 -> [il_dq]
  "abc -> dq (Power-Invariant)2"/1 -> [ig_dq]
  "abc -> dq (Power-Invariant)"/1 -> [vc_dq]
  [ig_abc] -> "Frequency Droop (iabc -> id)"/1(iabc)
  [il_dq] -> Current Controller/2(iIdq)
  [ig_dq] -> PQ Calculation (dq-Frame)/2
  PQ Calculation (dq-Frame)/1 -> [pq]
  [vc_dq] -> PQ Calculation (dq-Frame)/1
  [theta] -> "dq -> abc (Power-Invariant)"/2
  [vc_dq] -> Current Controller/3(vdq)
  Constant/1 -> Current Controller/4(enable)
  "Frequency Droop (iabc -> id)"/1(w) -> [w]
  "Frequency Droop (iabc -> id)"/2(theta) -> [theta]
  [theta] -> "abc -> dq (Power-Invariant)2"/2
  [ig_abc] -> "abc -> dq (Power-Invariant)2"/1
  [il_abc] -> "abc -> dq (Power-Invariant)1"/1
  [vc_abc] -> "abc -> dq (Power-Invariant)"/1
  [theta] -> "abc -> dq (Power-Invariant)1"/2
  [theta] -> "abc -> dq (Power-Invariant)"/2
  Demux/3 -> vc/1
  Demux/2 -> vb/1
  Demux/1 -> va/1
  LCL Filter/1(m) -> [m_filter]
  Bus Creator3/1 -> m/1
  "dq -> abc (Power-Invariant)"/1 -> [vi_abc]
  m_scale/1 -> "Frequency Droop (iabc -> id)"/2(m_scale)
  [vi_abc] -> Gain5/1
  Unit Delay/1 -> Demux/1
  Demux1/1 -> "Frequency Droop (iabc -> id)"/3(p)
  [pq] -> Demux1/1
  Bus Selector1/3 -> Gain4/1  "<igabc>"
  Bus Selector1/2 -> Gain3/1  "<ilabc>"
  Bus Selector1/1 -> Gain2/1  "<vcabc>"
  Gain4/1 -> [ig_abc]  "w"
  [m_filter] -> Bus Selector1/1
  Gain2/1 -> [vc_abc]  "w"
  Gain3/1 -> [il_abc]  "w"
  Gain5/1 -> Unit Delay/1  "w"
  Manual Switch1/1 -> [vi_dq], "dq -> abc (Power-Invariant)"/1
  Current Controller/1(vidq*) -> Manual Switch1/2
  connections:
  LCL Filter/LConn3 -- vc/RConn1
  va/LConn1 -- vb/LConn1 -- vc/LConn1 -- LCL Filter/LConn4 -- N/RConn1
  LCL Filter/RConn3 -- c/RConn1
  LCL Filter/RConn2 -- b/RConn1
  LCL Filter/RConn1 -- a/RConn1
  LCL Filter/LConn1 -- va/RConn1
  LCL Filter/LConn2 -- vb/RConn1

== system GFMGSP/Phase jump ==
  note: Pulse generator
      |
      | Author(s): Yitong Li
  Gain : Gain  Gain=Am
  Product : Product
  Step : Step  Time=t0  SampleTime=0
  Step1 : Step  Time=t0+dt  Before=1  After=0  SampleTime=0
  Out : Outport
  wires:
  Step1/1 -> Product/2
  Step/1 -> Product/1
  Product/1 -> Gain/1
  Gain/1 -> Out/1

== system GFMGSP/Phase jump1 ==
  note: Pulse generator
      |
      | Author(s): Yitong Li
  Gain : Gain  Gain=Am
  Product : Product
  Step : Step  Time=t0  SampleTime=0
  Step1 : Step  Time=t0+dt  Before=1  After=0  SampleTime=0
  Out : Outport
  wires:
  Step1/1 -> Product/2
  Step/1 -> Product/1
  Product/1 -> Gain/1
  Gain/1 -> Out/1

== system GFMGSP/Phase jump2 ==
  note: Pulse generator
      |
      | Author(s): Yitong Li
  Gain : Gain  Gain=Am
  Product : Product
  Step : Step  Time=t0  SampleTime=0
  Step1 : Step  Time=t0+dt  Before=1  After=0  SampleTime=0
  Out : Outport
  wires:
  Step1/1 -> Product/2
  Step/1 -> Product/1
  Product/1 -> Gain/1
  Gain/1 -> Out/1

== system GFMGSP/Voltage Sag ==
  note: Pulse generator
      |
      | Author(s): Yitong Li
  Constant : Constant
  Gain : Gain  Gain=1-Am
  Product : Product
  Step : Step  Time=t0  SampleTime=0
  Step1 : Step  Time=t0+dt  Before=1  After=0  SampleTime=0
  Subtract : Sum  Inputs=+-
  Out : Outport
  wires:
  Step1/1 -> Product/2
  Step/1 -> Product/1
  Product/1 -> Gain/1
  Gain/1 -> Subtract/2
  Subtract/1 -> Out/1
  Constant/1 -> Subtract/1

== system GFMGSP/Voltage Sag1 ==
  note: Pulse generator
      |
      | Author(s): Yitong Li
  Constant : Constant
  Gain : Gain  Gain=1-Am
  Product : Product
  Step : Step  Time=t0  SampleTime=0
  Step1 : Step  Time=t0+dt  Before=1  After=0  SampleTime=0
  Subtract : Sum  Inputs=+-
  Out : Outport
  wires:
  Step1/1 -> Product/2
  Step/1 -> Product/1
  Product/1 -> Gain/1
  Gain/1 -> Subtract/2
  Subtract/1 -> Out/1
  Constant/1 -> Subtract/1

== system GFMGSP/Voltage Sag2 ==
  note: Pulse generator
      |
      | Author(s): Yitong Li
  Constant : Constant
  Gain : Gain  Gain=1-Am
  Product : Product
  Step : Step  Time=t0  SampleTime=0
  Step1 : Step  Time=t0+dt  Before=1  After=0  SampleTime=0
  Subtract : Sum  Inputs=+-
  Out : Outport
  wires:
  Step1/1 -> Product/2
  Step/1 -> Product/1
  Product/1 -> Gain/1
  Gain/1 -> Subtract/2
  Subtract/1 -> Out/1
  Constant/1 -> Subtract/1

== system GFMGSP/abc -> dq (Power-Invariant)1 ==
  note: Frame transformation from abc to dq.
      |
      | Author(s): Yitong Li
      |
      | Notes:
      |
      | The transformation is power-invariant.
      |
      | theta is the angle that d axis leads a axis.
      |
      | q axis leads d axis by 90 degrees.
  abc : Inport
  theta : Inport  Port=2
  ->d : Fcn  Expr=cos(u(4))*u(1) + cos(u(4)-2/3*pi)*u(2) + cos(u(4)-4/3*pi)*u(3)
  ->q : Fcn  Expr=-sin(u(4))*u(1) - sin(u(4)-2/3*pi)*u(2) - sin(u(4)-4/3*pi)*u(3)
  Gain : Gain  Gain=sqrt(2/3)
  Mux5 : Mux  Inputs=2
  Mux6 : Mux  Inputs=2
  dq : Outport
  wires:
  abc/1 -> Gain/1
  ->d/1 -> Mux6/1
  Gain/1 -> Mux5/1
  theta/1 -> Mux5/2
  ->q/1 -> Mux6/2
  Mux6/1 -> dq/1
  Mux5/1 -> ->d/1, ->q/1

== system GFMGSP/abc -> dq (Power-Invariant)4 ==
  note: Frame transformation from abc to dq.
      |
      | Author(s): Yitong Li
      |
      | Notes:
      |
      | The transformation is power-invariant.
      |
      | theta is the angle that d axis leads a axis.
      |
      | q axis leads d axis by 90 degrees.
  abc : Inport
  theta : Inport  Port=2
  ->d : Fcn  Expr=cos(u(4))*u(1) + cos(u(4)-2/3*pi)*u(2) + cos(u(4)-4/3*pi)*u(3)
  ->q : Fcn  Expr=-sin(u(4))*u(1) - sin(u(4)-2/3*pi)*u(2) - sin(u(4)-4/3*pi)*u(3)
  Gain : Gain  Gain=sqrt(2/3)
  Mux5 : Mux  Inputs=2
  Mux6 : Mux  Inputs=2
  dq : Outport
  wires:
  abc/1 -> Gain/1
  ->d/1 -> Mux6/1
  Gain/1 -> Mux5/1
  theta/1 -> Mux5/2
  ->q/1 -> Mux6/2
  Mux6/1 -> dq/1
  Mux5/1 -> ->d/1, ->q/1

== system GFMGSP/enable ==
  note: Pulse generator
      |
      | Author(s): Yitong Li
  Gain : Gain
  Product : Product
  Step : Step  Time=t0  SampleTime=0
  Step1 : Step  Time=t0+dt  Before=1  After=0  SampleTime=0
  Out : Outport
  wires:
  Step1/1 -> Product/2
  Step/1 -> Product/1
  Product/1 -> Gain/1
  Gain/1 -> Out/1

== system GFMGSP/measurement1 ==
  Mux1 : Mux  Inputs=3
  Mux2 : Mux  Inputs=3
  ila : spsCurrentMeasurementLib/Current Measurement  PhasorSimulation=off  OutputType=Complex  PSBequivalent=0
  ilb : spsCurrentMeasurementLib/Current Measurement  PhasorSimulation=off  OutputType=Complex  PSBequivalent=0
  ilc : spsCurrentMeasurementLib/Current Measurement  PhasorSimulation=off  OutputType=Complex  PSBequivalent=0
  vca measure : spsVoltageMeasurementLib/Voltage Measurement  PhasorSimulation=off  OutputType=Complex  PSBequivalent=0
  vcb measure : spsVoltageMeasurementLib/Voltage Measurement  PhasorSimulation=off  OutputType=Complex  PSBequivalent=0
  vcc measure : spsVoltageMeasurementLib/Voltage Measurement  PhasorSimulation=off  OutputType=Complex  PSBequivalent=0
  a : PMIOPort  Side=Left
  b : PMIOPort  Port=2  Side=Left
  c : PMIOPort  Port=3  Side=Left
  n : PMIOPort  Port=4  Side=Left
  A : PMIOPort  Port=5  Side=Right
  B : PMIOPort  Port=6  Side=Right
  C : PMIOPort  Port=7  Side=Right
  N : PMIOPort  Port=8  Side=Right
  Iabc : Outport
  Vabc : Outport  Port=2
  wires:
  ila/1 -> Mux2/1
  ilb/1 -> Mux2/2
  ilc/1 -> Mux2/3
  Mux2/1 -> Iabc/1
  vcb measure/1 -> Mux1/2
  vca measure/1 -> Mux1/1
  vcc measure/1 -> Mux1/3
  Mux1/1 -> Vabc/1
  connections:
  a/RConn1 -- ila/LConn1
  ila/RConn1 -- A/RConn1 -- vca measure/LConn1
  ilb/LConn1 -- b/RConn1
  ilb/RConn1 -- B/RConn1 -- vcb measure/LConn1
  c/RConn1 -- ilc/LConn1
  C/RConn1 -- ilc/RConn1 -- vcc measure/LConn1
  n/RConn1 -- vcc measure/LConn2 -- vcb measure/LConn2 -- vca measure/LConn2 -- N/RConn1

== system GFMGSP/measurement10 ==
  Iabc : Inport
  Vabc : Inport  Port=2
  Complex to Magnitude-Angle : ComplexToMagnitudeAngle
  Demux1 : Demux  Outputs=2
  Demux2 : Demux  Outputs=2
  Divide : Product  Inputs=*/
  Gain : Gain  Gain=180/pi
  Real-Imag to Complex : RealImagToComplex
  Real-Imag to Complex1 : RealImagToComplex
  "abc -> dq (Power-Invariant)1" : Subsystem  AncestorBlock=|
      | SimplusGT/abc -> dq
      | (Power-Invariant)
  "abc -> dq (Power-Invariant)4" : Subsystem  AncestorBlock=|
      | SimplusGT/abc -> dq
      | (Power-Invariant)
  phi : Outport
  Zm : Outport  Port=2
  wires:
  Vabc/1 -> "abc -> dq (Power-Invariant)4"/1(abc)
  [theta2G] -> "abc -> dq (Power-Invariant)4"/2(theta), "abc -> dq (Power-Invariant)1"/2(theta)
  Iabc/1 -> "abc -> dq (Power-Invariant)1"/1(abc)
  "abc -> dq (Power-Invariant)4"/1(dq) -> Demux1/1
  Demux1/1 -> Real-Imag to Complex/1
  Demux1/2 -> Real-Imag to Complex/2
  Demux2/1 -> Real-Imag to Complex1/1
  Demux2/2 -> Real-Imag to Complex1/2
  "abc -> dq (Power-Invariant)1"/1(dq) -> Demux2/1
  Real-Imag to Complex/1 -> Divide/1
  Real-Imag to Complex1/1 -> Divide/2
  Divide/1 -> Complex to Magnitude-Angle/1
  Complex to Magnitude-Angle/1 -> Zm/1
  Gain/1 -> phi/1
  Complex to Magnitude-Angle/2 -> Gain/1

== system GFMGSP/measurement11 ==
  Iabc : Inport
  Vabc : Inport  Port=2
  Complex to Magnitude-Angle : ComplexToMagnitudeAngle
  Demux1 : Demux  Outputs=2
  Demux2 : Demux  Outputs=2
  Divide : Product  Inputs=*/
  Gain : Gain  Gain=180/pi
  Real-Imag to Complex : RealImagToComplex
  Real-Imag to Complex1 : RealImagToComplex
  "abc -> dq (Power-Invariant)1" : Subsystem  AncestorBlock=|
      | SimplusGT/abc -> dq
      | (Power-Invariant)
  "abc -> dq (Power-Invariant)4" : Subsystem  AncestorBlock=|
      | SimplusGT/abc -> dq
      | (Power-Invariant)
  phi : Outport
  Zm : Outport  Port=2
  wires:
  Vabc/1 -> "abc -> dq (Power-Invariant)4"/1(abc)
  [theta2G] -> "abc -> dq (Power-Invariant)4"/2(theta), "abc -> dq (Power-Invariant)1"/2(theta)
  Iabc/1 -> "abc -> dq (Power-Invariant)1"/1(abc)
  "abc -> dq (Power-Invariant)4"/1(dq) -> Demux1/1
  Demux1/1 -> Real-Imag to Complex/1
  Demux1/2 -> Real-Imag to Complex/2
  Demux2/1 -> Real-Imag to Complex1/1
  Demux2/2 -> Real-Imag to Complex1/2
  "abc -> dq (Power-Invariant)1"/1(dq) -> Demux2/1
  Real-Imag to Complex/1 -> Divide/1
  Real-Imag to Complex1/1 -> Divide/2
  Divide/1 -> Complex to Magnitude-Angle/1
  Complex to Magnitude-Angle/1 -> Zm/1
  Gain/1 -> phi/1
  Complex to Magnitude-Angle/2 -> Gain/1

== system GFMGSP/measurement12 ==
  Iabc : Inport
  Vabc : Inport  Port=2
  Complex to Magnitude-Angle : ComplexToMagnitudeAngle
  Demux1 : Demux  Outputs=2
  Demux2 : Demux  Outputs=2
  Divide : Product  Inputs=*/
  Gain : Gain  Gain=180/pi
  Real-Imag to Complex : RealImagToComplex
  Real-Imag to Complex1 : RealImagToComplex
  "abc -> dq (Power-Invariant)1" : Subsystem  AncestorBlock=|
      | SimplusGT/abc -> dq
      | (Power-Invariant)
  "abc -> dq (Power-Invariant)4" : Subsystem  AncestorBlock=|
      | SimplusGT/abc -> dq
      | (Power-Invariant)
  phi : Outport
  Zm : Outport  Port=2
  wires:
  Vabc/1 -> "abc -> dq (Power-Invariant)4"/1(abc)
  [theta2G] -> "abc -> dq (Power-Invariant)4"/2(theta), "abc -> dq (Power-Invariant)1"/2(theta)
  Iabc/1 -> "abc -> dq (Power-Invariant)1"/1(abc)
  "abc -> dq (Power-Invariant)4"/1(dq) -> Demux1/1
  Demux1/1 -> Real-Imag to Complex/1
  Demux1/2 -> Real-Imag to Complex/2
  Demux2/1 -> Real-Imag to Complex1/1
  Demux2/2 -> Real-Imag to Complex1/2
  "abc -> dq (Power-Invariant)1"/1(dq) -> Demux2/1
  Real-Imag to Complex/1 -> Divide/1
  Real-Imag to Complex1/1 -> Divide/2
  Divide/1 -> Complex to Magnitude-Angle/1
  Complex to Magnitude-Angle/1 -> Zm/1
  Gain/1 -> phi/1
  Complex to Magnitude-Angle/2 -> Gain/1

== system GFMGSP/measurement13 ==
  Iabc : Inport
  Vabc : Inport  Port=2
  Complex to Magnitude-Angle : ComplexToMagnitudeAngle
  Demux1 : Demux  Outputs=2
  Demux2 : Demux  Outputs=2
  Divide : Product  Inputs=*/
  Gain : Gain  Gain=180/pi
  Real-Imag to Complex : RealImagToComplex
  Real-Imag to Complex1 : RealImagToComplex
  "abc -> dq (Power-Invariant)1" : Subsystem  AncestorBlock=|
      | SimplusGT/abc -> dq
      | (Power-Invariant)
  "abc -> dq (Power-Invariant)4" : Subsystem  AncestorBlock=|
      | SimplusGT/abc -> dq
      | (Power-Invariant)
  phi : Outport
  Zm : Outport  Port=2
  wires:
  Vabc/1 -> "abc -> dq (Power-Invariant)4"/1(abc)
  [theta2G] -> "abc -> dq (Power-Invariant)4"/2(theta), "abc -> dq (Power-Invariant)1"/2(theta)
  Iabc/1 -> "abc -> dq (Power-Invariant)1"/1(abc)
  "abc -> dq (Power-Invariant)4"/1(dq) -> Demux1/1
  Demux1/1 -> Real-Imag to Complex/1
  Demux1/2 -> Real-Imag to Complex/2
  Demux2/1 -> Real-Imag to Complex1/1
  Demux2/2 -> Real-Imag to Complex1/2
  "abc -> dq (Power-Invariant)1"/1(dq) -> Demux2/1
  Real-Imag to Complex/1 -> Divide/1
  Real-Imag to Complex1/1 -> Divide/2
  Divide/1 -> Complex to Magnitude-Angle/1
  Complex to Magnitude-Angle/1 -> Zm/1
  Gain/1 -> phi/1
  Complex to Magnitude-Angle/2 -> Gain/1

== system GFMGSP/measurement14 ==
  Iabc : Inport
  Vabc : Inport  Port=2
  Complex to Magnitude-Angle : ComplexToMagnitudeAngle
  Demux1 : Demux  Outputs=2
  Demux2 : Demux  Outputs=2
  Divide : Product  Inputs=*/
  Gain : Gain  Gain=180/pi
  Real-Imag to Complex : RealImagToComplex
  Real-Imag to Complex1 : RealImagToComplex
  "abc -> dq (Power-Invariant)1" : Subsystem  AncestorBlock=|
      | SimplusGT/abc -> dq
      | (Power-Invariant)
  "abc -> dq (Power-Invariant)4" : Subsystem  AncestorBlock=|
      | SimplusGT/abc -> dq
      | (Power-Invariant)
  phi : Outport
  Zm : Outport  Port=2
  wires:
  Vabc/1 -> "abc -> dq (Power-Invariant)4"/1(abc)
  [theta2G] -> "abc -> dq (Power-Invariant)4"/2(theta), "abc -> dq (Power-Invariant)1"/2(theta)
  Iabc/1 -> "abc -> dq (Power-Invariant)1"/1(abc)
  "abc -> dq (Power-Invariant)4"/1(dq) -> Demux1/1
  Demux1/1 -> Real-Imag to Complex/1
  Demux1/2 -> Real-Imag to Complex/2
  Demux2/1 -> Real-Imag to Complex1/1
  Demux2/2 -> Real-Imag to Complex1/2
  "abc -> dq (Power-Invariant)1"/1(dq) -> Demux2/1
  Real-Imag to Complex/1 -> Divide/1
  Real-Imag to Complex1/1 -> Divide/2
  Divide/1 -> Complex to Magnitude-Angle/1
  Complex to Magnitude-Angle/1 -> Zm/1
  Gain/1 -> phi/1
  Complex to Magnitude-Angle/2 -> Gain/1

== system GFMGSP/measurement15 ==
  Iabc : Inport
  Vabc : Inport  Port=2
  Complex to Magnitude-Angle : ComplexToMagnitudeAngle
  Demux1 : Demux  Outputs=2
  Demux2 : Demux  Outputs=2
  Divide : Product  Inputs=*/
  Filter p : DiscreteTransferFcn  Numerator=10*2*pi*Ts  Denominator=[1 ((10*2*pi*Ts)-1)]  SampleTime=Ts
  Filter p1 : DiscreteTransferFcn  Numerator=10*2*pi*Ts  Denominator=[1 ((10*2*pi*Ts)-1)]  SampleTime=Ts
  Gain : Gain  Gain=180/pi
  Real-Imag to Complex : RealImagToComplex
  Real-Imag to Complex1 : RealImagToComplex
  Scope27 : Scope  NumInputPorts=4
  "abc -> dq (Power-Invariant)1" : Subsystem  AncestorBlock=|
      | SimplusGT/abc -> dq
      | (Power-Invariant)
  "abc -> dq (Power-Invariant)4" : Subsystem  AncestorBlock=|
      | SimplusGT/abc -> dq
      | (Power-Invariant)
  phi : Outport
  Zm : Outport  Port=2
  wires:
  Vabc/1 -> "abc -> dq (Power-Invariant)4"/1(abc)
  [theta2G] -> "abc -> dq (Power-Invariant)4"/2(theta), "abc -> dq (Power-Invariant)1"/2(theta)
  Iabc/1 -> "abc -> dq (Power-Invariant)1"/1(abc)
  "abc -> dq (Power-Invariant)4"/1(dq) -> Scope27/1, Filter p/1
  Demux1/1 -> Real-Imag to Complex/1
  Demux1/2 -> Real-Imag to Complex/2
  Demux2/1 -> Real-Imag to Complex1/1
  Demux2/2 -> Real-Imag to Complex1/2
  "abc -> dq (Power-Invariant)1"/1(dq) -> Scope27/3, Filter p1/1
  Real-Imag to Complex/1 -> Divide/1
  Real-Imag to Complex1/1 -> Divide/2
  Divide/1 -> Complex to Magnitude-Angle/1
  Complex to Magnitude-Angle/1 -> Zm/1
  Gain/1 -> phi/1
  Complex to Magnitude-Angle/2 -> Gain/1
  Filter p/1 -> Scope27/2, Demux1/1
  Filter p1/1 -> Scope27/4, Demux2/1

== system GFMGSP/measurement16 ==
  Iabc : Inport
  Vabc : Inport  Port=2
  Complex to Magnitude-Angle : ComplexToMagnitudeAngle
  Demux1 : Demux  Outputs=2
  Demux2 : Demux  Outputs=2
  Divide : Product  Inputs=*/
  Gain : Gain  Gain=180/pi
  Real-Imag to Complex : RealImagToComplex
  Real-Imag to Complex1 : RealImagToComplex
  "abc -> dq (Power-Invariant)1" : Subsystem  AncestorBlock=|
      | SimplusGT/abc -> dq
      | (Power-Invariant)
  "abc -> dq (Power-Invariant)4" : Subsystem  AncestorBlock=|
      | SimplusGT/abc -> dq
      | (Power-Invariant)
  phi : Outport
  Zm : Outport  Port=2
  wires:
  Vabc/1 -> "abc -> dq (Power-Invariant)4"/1(abc)
  [theta2G] -> "abc -> dq (Power-Invariant)4"/2(theta), "abc -> dq (Power-Invariant)1"/2(theta)
  Iabc/1 -> "abc -> dq (Power-Invariant)1"/1(abc)
  "abc -> dq (Power-Invariant)4"/1(dq) -> Demux1/1
  Demux1/1 -> Real-Imag to Complex/1
  Demux1/2 -> Real-Imag to Complex/2
  Demux2/1 -> Real-Imag to Complex1/1
  Demux2/2 -> Real-Imag to Complex1/2
  "abc -> dq (Power-Invariant)1"/1(dq) -> Demux2/1
  Real-Imag to Complex/1 -> Divide/1
  Real-Imag to Complex1/1 -> Divide/2
  Divide/1 -> Complex to Magnitude-Angle/1
  Complex to Magnitude-Angle/1 -> Zm/1
  Gain/1 -> phi/1
  Complex to Magnitude-Angle/2 -> Gain/1
